simulink model "pp_c_tf"  (Simulink 5.0)
settings: Solver=ode23s  StartTime=t0  StopTime=tf  RelTol=1e-8  AbsTol=1.0e-8
values from neighbouring files (symbols this model uses):
  den = poly([-143 -162+30*j -162-30*j -30+15*j -30-15*j -21+6*j -21-6*j])    [roll_im.m]    (also in sigurd.m = conv([10 1],den); unstb2.m = conv([1 -3],[1 2]))
  num = 26.24*poly([-190 -21+11*j -21-11*j -20 -0.5+86*j -0.5-86*j])    [roll_im.m]    (also in sigurd.m = 200; unstb2.m = [1 -1])
  R = 9.76e-4*[1 -0.5625]    [pplace2.m]
  S = 0.1426    [pplace2.m]
  st = 1    [ant.m]    (also in dof_choice.m; motor.m; roll_im.m = 0.2; sigurd.m)
  Ts = 0.2; [B,A,k] = myc2d(G,Ts)    [ant.m]    (also in dof_choice.m = 1; motor.m = 0.25; [B,A,k] = myc2d(G,Ts); roll_im.m = 0.001; sigurd.m = 0.025)
undefined symbols (not defined in the file or in its folder): tau, TM
settings Model: Creator=kannanm  LastModifiedBy=kannan  ExtModeAutoUpdateStatusClock=off

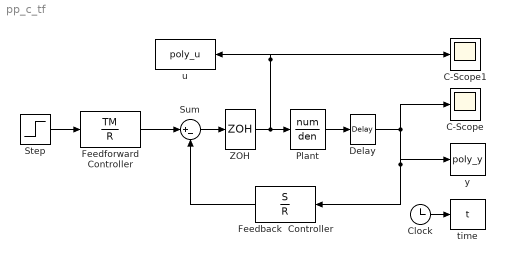
== system pp_c_tf ==
  C-Scope : Scope
      settings: YMin=-5e+13  YMax=4e+14
  C-Scope1 : Scope
      settings: YMin=-3e+14  YMax=3e+14
  Clock : Clock
      settings: Decimation=10
  Delay : TransportDelay  DelayTime=tau
  Feedback  Controller : DiscreteFilter  Orientation=left  Numerator=S  Denominator=R  SampleTime=Ts
  Feedforward Controller : DiscreteFilter  Numerator=TM  Denominator=R  SampleTime=Ts
  Plant : TransferFcn  Numerator=num  Denominator=den
  Step : Step  Time=0  After=st  SampleTime=Ts
  Sum : Sum  Inputs=|+-  SaturateOnIntegerOverflow=on
  ZOH : ZeroOrderHold  SampleTime=Ts
  time : ToWorkspace  VariableName=t  SampleTime=Ts  SaveFormat=Array
  u : ToWorkspace  VariableName=poly_u  SampleTime=Ts  SaveFormat=Array
  y : ToWorkspace  VariableName=poly_y  SampleTime=Ts  SaveFormat=Array
  wires:
  Step/1 -> Feedforward Controller/1
  Feedforward Controller/1 -> Sum/1
  Sum/1 -> ZOH/1
  Feedback  Controller/1 -> Sum/2
  ZOH/1 -> Plant/1, u/1, C-Scope1/1
  Clock/1 -> time/1
  Plant/1 -> Delay/1
  Delay/1 -> C-Scope/1, Feedback  Controller/1, y/1
